simulink library "vectorMagnitude_ul"  (R2020a)
settings: Solver=VariableStepAuto  StartTime=0.0  StopTime=10.0  RelTol=1e-3
settings Model: Creator=JohnJr  LastModifiedBy=JohnJr

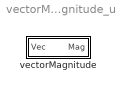
== system vectorMagnitude_ul ==
  vectorMagnitude : Subsystem

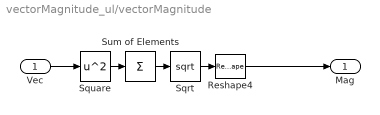
== system vectorMagnitude_ul/vectorMagnitude ==
  Vec : Inport
  Reshape4 : Reshape
  Sqrt : Sqrt  SaturateOnIntegerOverflow=on
  Square : Math  Operator=square  SaturateOnIntegerOverflow=on
  Sum of Elements : Sum  Inputs=+
  Mag : Outport
  wires:
  Sqrt/1 -> Reshape4/1
  Square/1 -> Sum of Elements/1
  Sum of Elements/1 -> Sqrt/1
  Vec/1 -> Square/1
  Reshape4/1 -> Mag/1
